simulink model "CD2_Library"  (Simulink 8.6)
settings: Solver=FixedStepDiscrete  StartTime=0  StopTime=7200  FixedStep=300  RelTol=1e-3
InitFcn:
  | CD2_init
undefined symbols (not defined in the file): CD2_get_substance_count, CD2_get_substances_count, Crain, get_blocks_id, input_c, subs_vect, table, tablestep
(part 1 of 2)
settings Model: Creator=garbanlo  LastModifiedBy=garbanlo
settings DataIOCC: LimitDataPoints=off  TimeSaveName=cd_time  SignalLoggingName=sigsOut
settings OptimizationCC: ExpressionDepthLimit=128  InitFltsAndDblsToZero=on
settings DebuggingCC: SaveWithParameterizedLinksMsg=none  SignalResolutionControl=TryResolveAllWithWarning  SolverPrmCheckMsg=none  MultiTaskDSMMsg=warning  MultiTaskCondExecSysMsg=none  FcnCallInpInsideContextMsg=UseLocalSettings  StateNameClashWarn=none  StrictBusMsg=None
settings HardwareCC: TargetUnknown=on
settings GRTTargetCC: TargetFcnLib=ansi_tfl_tmw.mat  GeneratePreprocessorConditionals=Use local settings

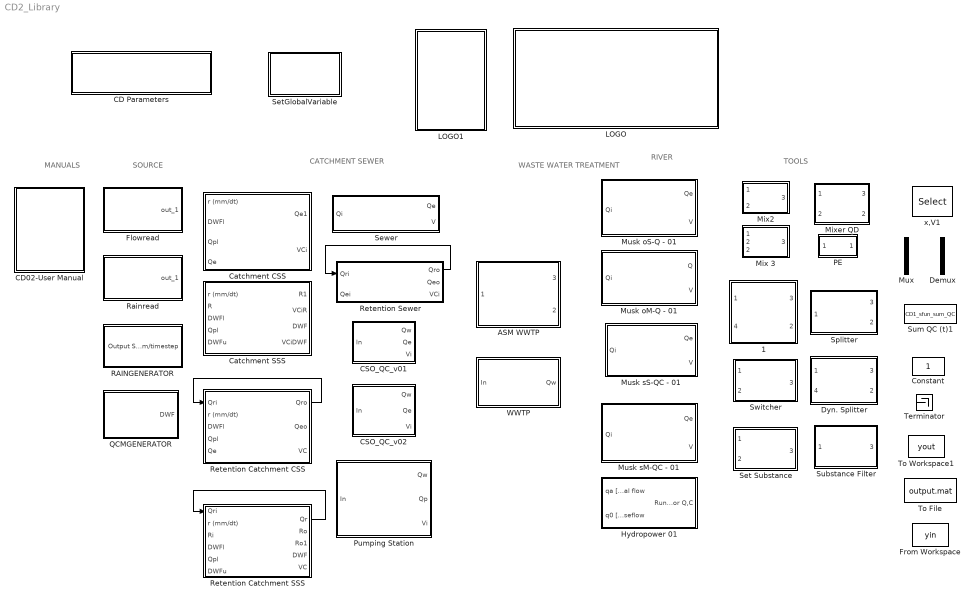
== system CD2_Library ==
  note: TOOLS
  note: SOURCE
  note: RIVER
  note: CATCHMENT
      | SEWER
  note: MANUALS
  note: WASTE WATER
      | TREATMENT
  " 1" : Subsystem  mask(Wrong Connect){n_comp=CD2_get_substances_count, values_rain=15, mode_rain=Percent [0-100], values_dwf=23, mode_dwf=Percent [0-100]}
      mask prompts: n_comp "Number of components"; values_rain "Fraction Qr --> Qdwf"; mode_rain "Splitting mode"; values_dwf "Fraction Qdwf --> Qr"; mode_dwf "Splitting mode"
      mask help: The block simulates wrong connections given in a seperate sewer system. MAgnitudes of wrong connections are described by fraction percentages (or quanities) diverted from or to the stormwater pipe.
      mask init:
      | % reading the toplevel systems' name 
      | % --> Plant file name;
      | tls=bdroot(gcb); 
      | % Obtaining the fixed sampling time
      | t_samp_char=get_param(tls, 'FixedStep');
      | % Convertion to numeric value
      | tstep = str2num(t_samp_char);
      mask TypeOptions mode_rain: Fraction [0-1] | Percent [0-100] | m³/s
      mask TypeOptions mode_dwf: Fraction [0-1] | Percent [0-100] | m³/s
      mask Display:
      | plot(0,0,100,100);
      | 
      | 
      | plot([30,70],[30,30]);
      | plot([30,70],[70,70]);
      | plot([40,60],[30,70]);
      | plot([40,60],[70,30]);
      | 
      | 
      | 
      | 
      | text(50,10,'WRONG Connect','HorizontalAlignment','center');
      | port_label('input',1,'Qr');
      | port_label('input',2,'Qdwf');
      | port_label('output',1,'Qr');
      | port_label('output',2,'Qdwf');
  " Dyn. Splitter" : Subsystem  mask(Splitter){n_comp=CD2_get_substances_count, mode=Percent [0-100]}
      mask prompts: n_comp "Number of components"; mode "Splitting mode"
      mask help: Splitter parameter.
      mask init: same as CD2_Library/ 1
      mask Help: Splits stream in 2 streams. Split by percent or by value.
      mask TypeOptions mode: Fraction [0-1] | Percent [0-100] | m³/s
      mask Display:
      | plot(0,0,100,100);
      | 
      | plot([30,50],[50,50]);
      | plot([50,70],[50,70]);
      | plot([50,70],[50,30]);
      | 
      | text(50,10,'Dyn. SPLITTER','HorizontalAlignment','center');
      | port_label('input',1,'Qi');
      | port_label('output',1,'Q1');
      | port_label('output',2,'Q2');
  " Hydropower 01" : Subsystem  mask(HYDROPOWER){n_comp=CD2_get_substances_count, C_Stream=[1 2 3]}
      mask prompts: n_comp "No of components"; C_Stream "Vector of Stream-Conc. g/m3"
      mask help:
      | Hydropower block for modelling downstream release of water. Upstream concnetration of baseflow ( qo ) and additional flow ( qa ) are considered constant.
      |
      | Used function:
      | CD1_sfun_hydropower
      mask init:
      | % reading the toplevel systems' name 
      | % --> Plant file name;
      | tls=bdroot(gcb); 
      | % Obtaining the fixed sampling time
      | t_samp_char=get_param(tls, 'FixedStep');
      | % Convertion to numeric value
      | tstep = str2num(t_samp_char);
      mask Display:
      | plot(0,0,100,100, [30 30 32 34 36 38 40 44 46 50], [28 60 62 65 67 70 70 67 65 25], [15 80],[30 20], [30 50],[34 30],[30 50],[38 34], [15 33],[65 65], [50 80],[45 40] );
      | text(50,90,'HYDROPOWER','HorizontalAlignment','center');
      | text(50,10,'baseflow','HorizontalAlignment','center');
      | port_label('input',1,'qa');
      | port_label('input',2,'qo');
      | port_label('output',1,'Qe');
  " Mixer QD" : Subsystem  mask(Mixer QD){n_comp=CD2_get_substances_count, Cmcl=[3 3 3]}
      mask prompts: n_comp "Number of pollutants [ - ]"; Cmcl "MCL - Vector of max. concentration limits [g/m3]"
      mask help:
      | Performes mixing of pollutant fluxes Qw  and Qo in accordance to their hydraulic load. Qo is considered to be the less pollluted flux. In addition the required increase of Qo is calculated for meeting required MCL (maximum concentration limits) defined by user input.
      |
      | Function used:
      | CD1_sfun_mixing_QC_QD.m
      mask init: same as CD2_Library/ 1
      mask Display:
      | plot(0,0,100,100);
      | 
      | text(50,60,'Mixing','HorizontalAlignment','center');
      | text(50,35,'QD','HorizontalAlignment','center');
      | 
      | 
      | port_label('input',1,'Qw');
      | port_label('input',2,'Qo');
      | port_label('output',1,'Qe');
      | port_label('output',2,'QD');
  ASM WWTP : Subsystem  mask(ASM WWTP){wwtpfile='wwtp_vils.txt', dtwwtp=30, frac=[1 1 1], n_comp=CD2_get_substances_count}
      mask prompts: wwtpfile "WWTP File"; dtwwtp "delta t WWTP"; frac "Fraction sol [0-1]"; n_comp "Number of pollutants [ - ]"
      mask help: WWTP unit that includes primray clarifier, biology and secondary clarifier. Biochemical modelling is based on a simplified ASM1 model.
      mask init: same as CD2_Library/ 1
      mask Display:
      | plot(0,0,100,100);
      | 
      | plot(0,0,100,100);
      | 
      | patch( [15,35,25,15],[55,55,30,55],[.6 0.6 .3]);
      | patch( [40,60,60,40,40],[30,30,55,55,30],[.8 0.6 .3]);
      | patch( [65,85,75,65],[55,55,30,55],[1 0.6 .3]);
      | 
      | plot( [15,35,25,15],[55,55,30,55], [30, 40],[40,40], [40,60,60,40,40],[30,30,55,55,30], [65,85,75,65],[55,55,30,55], [60, 70],[40,40] );
      | 
      | 
      | 
      | text(50,70,'ASM-WWTP','HorizontalAlignment','center');
      | 
      | 
      | port_label('input',1,'Qi');
      | port_label('output',1,'Qe');
      | port_label('output',2,'ASM1+P');
  CD Parameters : Subsystem  mask(City Drain 2.0 - Simulation parameters){subst='HCO3 NH4', t_step=300, t_start=0, t_stop=7200}
      mask prompts: subst "Modell Substances list (string)"; t_step "Sampling Time [s]"; t_start "Start Time [s]"; t_stop "Stop Time [s]"
      mask help:
      | Block that sets the global parameters required in City Drain 2.0. Following paramters are set without user's input:
      |
      | - 'Solver' --> 'FixedStepDiscrete'
      | - 'TimeSaveName' --> 'cd_time'
      | - 'Decimation' --> '1'
      | - 'LimitDataPoints' -->  'off'
      mask init:
      | % toplevel systems' name --> Plant file name;
      | tls=bdroot(gcb); 
      | set_param(tls, 'Solver', 'FixedStepDiscrete'); 
      | set_param(tls, 'TimeSaveName', 'cd_time');
      | set_param(tls, 'Decimation', '1');
      | set_param(tls, 'LimitDataPoints', 'off');
      | set_param(tls, 'ScreenColor', 'white');
      | 
      | tstep_char=num2str(t_step); % Setting the discrete time step
      | set_param(tls, 'FixedStep', tstep_char); 
      | 
      | tstart_char=num2str(t_start); % Setting the start time
      | set_param(tls, 'StartTime', tstart_char); 
      | 
      | tstop_char=num2str(t_stop); % Setting the stop time
      | set_param(tls, 'StopTime', tstop_char);
      | 
      | set_param(gcs,'InitFcn','CD2_init');
      mask Display:
      | plot(0,0,100,100);
      | 
      | text(50,65,'CITY DRAIN','HorizontalAlignment','center');
      | text(50,35,'PARAMETERS','HorizontalAlignment','center');
      | 
      | 
      | image(imread('CityDrain_SimParam.jpg'))
  CD02-User Manual : Subsystem  mask(Open Usermanual){}
      settings: OpenFcn=open('CD2_UserManual_2007.pdf');
      mask Display:
      | text(50,70,'CITY DRAIN 1.0','HorizontalAlignment','center');
      | text(50,40,'User Manual','HorizontalAlignment','center');
      | image(imread('CD1_start_user_manual.jpg'));
  CSO_QC_v01 : Subsystem  mask(CSO Typ A - Combined sewer overflow){Vmax=300, Qemax=0.1, n_comp=CD2_get_substances_count}
      mask prompts: Vmax "Basin Volume [m3]"; Qemax "Maximum Effluent flow [m3/s]"; n_comp "Number of Pollutants [-]"
      mask help:
      | Combined sewer overflow structure.
      | Diverts the inflow given into effluent and overflow. The model implemented consideres hydraulics and pollutant routing by full mixing in the structure.
      |
      | Function used:
      | CD1_sfun_cso_A.m
      mask init: same as CD2_Library/ 1
      mask Display:
      | plot(0,0,100,100);
      | 
      | text(50,60,'CSO','HorizontalAlignment','center');
      | text(50,30,'Typ A','HorizontalAlignment','center');
      | 
      | 
      | port_label('input',1,'Qi');
      | port_label('output',1,'Qw');
      | port_label('output',2,'Qe');
      | port_label('output',3,'Vi');
  CSO_QC_v02 : Subsystem  mask(CSO Typ B - Combined sewer overflow){Vmax=300, Qemax=0.1, n_comp=CD2_get_substances_count, n_sed=[0.2]}
      mask prompts: Vmax "Basin Volume (m3)"; Qemax "Maximum Effluent flow [m3/s]"; n_comp "Number of Pollutants [-]"; n_sed "n-sed (Vect. of Sed. Coefficients)"
      mask help:
      | Combined sewer overflow structure.
      | Diverts the inflow given into effluent and overflow. The model implemented consideres hydraulics and pollutant routing by full mixing in the structure.
      |
      | In addition to Type A a retenetion/sedimentation factor is introduced. The factor may be used for applying different ratios in pollutant concentration for effluent flow (QE) and overflow (QW).
      |
      | Function used:
      | CD1_sfun_cso_B.m
      mask init: same as CD2_Library/ 1
      mask Display:
      | plot(0,0,100,100);
      | 
      | 
      | text(50,60,'CSO','HorizontalAlignment','center');
      | text(50,30,'Typ B','HorizontalAlignment','center');
      | 
      | 
      | port_label('input',1,'Qi');
      | port_label('output',1,'Qw');
      | port_label('output',2,'Qe');
      | port_label('output',3,'Vi');
  Catchment CSS : Subsystem  mask(Catchment CSS){area=208, rfcoeff=0.20, initloss=1, permloss=1.25, N=3, n_comp=CD2_get_substances_count, Rain_C=1, K=300, X=0}
      mask prompts: area "Area in [ha]"; rfcoeff "Runoff coefficient (0 - 1)"; initloss "Initial Loss in [mm]"; permloss "Permanent loss in [mm/day]"; N "No of Timesteps (transport time) / No of subareas n [-]"; n_comp "No of pollutant components"; Rain_C "Vector of Rain-Conc. [g/m3]"
      mask help:
      | Hydrological model of an urban catchment with a combined sewer system.
      | --> see manual for more details
      mask init:
      | % location of catchment drawing
      | x=10;
      | y=-10;
      | % reading the toplevel systems' name 
      | % --> Plant file name;
      | tls=bdroot(gcb); 
      | % Obtaining the fixed sampling time
      | t_samp_char=get_param(tls, 'FixedStep');
      | % Convertion to numeric value
      | tstep = str2num(t_samp_char); 
      | 
      | %convertion form mm/day --> mm/DT
      | permloss=permloss/86400*tstep;
      | area=area*10000;
      | 
      | %parameter for muskingum
      | CX=(tstep/2-K*X)/(tstep/2+K*(1-X));
      | CY=1/(tstep/2+K*(1-X));
      mask Display:
      | plot(0,0,100,100, [17 20 25 30 40 45 50 55 60 65]+x, [60 80 82 85 88 88 88 85 75 60]+y);
      | plot(0,0,100,100, [17 20 25 30 40 45 50 55 60 65]+x, [55 40 35 30 30 30 30 35 40 55]+y);
      | 
      | plot([20 65]+x,[60 60]+y);
      | plot([20 30]+x,[80 60]+y);
      | plot([30 40]+x,[75 60]+y);
      | plot([45 60]+x,[75 60]+y);
      | plot([20 65]+x,[55 55]+y);
      | plot([20 30]+x,[40 55]+y);
      | plot([30 40]+x,[45 55]+y);
      | plot([45 60]+x,[30 55]+y);
      | 
      | color('black');
      | 
      | port_label('input',1,'rl');
      | port_label('input',2,'DWFl');
      | port_label('input',3,'Qpl');
      | port_label('input',4,'Qe');
      | port_label('output',1,'Qe');
      | port_label('output',2,'VCi');
      | 
      | text(50,90,'CATCHMENT CSS','HorizontalAlignment','center');
  Catchment SSS : Subsystem  mask(Catchment SSS){area=27, rfcoeff=0.16, initloss=1, permloss=1.25, N=6, n_comp=CD2_get_substances_count, Rain_C=1, K=300, X=0}
      mask prompts: area "Area in [ha]"; rfcoeff "Runoff coefficient (0 - 1)"; initloss "Initial Loss in [mm]"; permloss "Permanent loss in [mm/day]"; N "No of Timesteps (transport time) / No of subareas n [-]"; n_comp "No of pollutant components"; Rain_C "Vector of Rain-Conc. [g/m3]"
      mask help:
      | Hydrological model of an urban catchment with a separate sewer system.
      | --> see manual for more details
      mask init: same as CD2_Library/Catchment CSS
      mask Display:
      | plot(0,0,100,100, [17 20 25 30 40 50 55 60 70 75 80]+x, [60 80 82 85 88 88 88 85 82 75 60]+y);
      | 
      | plot([20 80]+x,[60 60]+y);
      | plot([20 30]+x,[80 60]+y);
      | plot([30 40]+x,[75 60]+y);
      | plot([45 60]+x,[75 60]+y);
      | 
      | color('white');
      | plot([20 80]+x,[55 55]+y);
      | plot([20 30]+x,[40 55]+y);
      | plot([30 40]+x,[45 55]+y);
      | plot([45 60]+x,[30 55]+y);
      | 
      | color('black');
      | 
      | port_label('input',1,'rl');
      | port_label('input',2,'R');
      | port_label('input',3,'DWFl');
      | port_label('input',4,'Qpl');
      | port_label('input',5,'DWFu');
      | port_label('output',1,'R');
      | port_label('output',2,'VCi(R)');
      | port_label('output',3,'DWF');
      | port_label('output',4,'VCi(DWF)');
      | 
      | 
      | text(50,90,'CATCHMENT SSS','HorizontalAlignment','center');
  Constant : Constant
  Demux : Demux  Outputs=[13,1]
  Flowread : Subsystem  mask(CD1_Flowread){table0='Input_CSO_QC_Test_01.txt', dtype=Composite sample, crep=off}
      mask prompts: table0 "Filename"; dtype "Data type"; crep "Cylic repitition"
      mask help:
      | Reads flowdata (Q) and substance concentration (Ci) associated from ascii file.
      |
      | Used function:
      | CD1_sfun_flowread.m
      | CD1_mfun_flowread.m
      mask init:
      | table=CD1_mfun_flowread(table0);
      | 
      | 
      | % reading the toplevel systems' name 
      | % --> Plant file name;
      | tls=bdroot(gcb); 
      | % Obtaining the fixed sampling time
      | t_samp_char=get_param(tls, 'FixedStep');
      | % Convertion to numeric value
      | tstep = str2num(t_samp_char);
      mask TypeOptions dtype: Composite sample | Grab sample
      mask Display:
      | plot(0,0,100,100);
      | 
      | text(50,20,'FLOWREAD','HorizontalAlignment','center');
      | 
      | plot( [5 10 10 15 15 20 20 25 25 30 30 35 35 40], [0 0 10 10 20 20 40 40 20 20 0 0 0 0]+50);
      | plot( [5 10 15 20 25 30 35 ]+50, [0 5 10 15 30 20 0]+50);
  From Workspace : FromWorkspace  VariableName=yin  OutputAfterFinalValue=Setting to zero
  LOGO : Subsystem  mask(LOGO CITY DRAIN){}
      mask help:
      | Displays the City Drain Logo in Color
      |
      | Source file:
      | CityDrainLogo_C1.jpg
      mask Display: image(imread('CityDrain 2Logo_C1.jpg'));
  LOGO1 : Subsystem  mask(LOGO CITY DRAIN){}
      mask help:
      | Displays the City Drain Logo in Color
      |
      | Source file:
      | CityDrainLogo_C1.jpg
      mask Display: image(imread('LOGO_IUT4C.jpg'));
  Mix 3 : Subsystem  mask(Mixer){n_comp=CD2_get_substances_count}
      mask prompts: n_comp "Number of pollutants [ - ]"
      mask help:
      | Performes mixing of pollutant fluxes Q1 and Q2 in accordance to their hydraulic load.
      |
      | Function used:
      | CD1_sfun_mixing_QC.m
      mask init: same as CD2_Library/ 1
      mask Display:
      | plot(0,0,100,100);
      | 
      | text(50,50,'Mix3','HorizontalAlignment','center');
      | 
      | 
      | port_label('input',1,'Q1');
      | port_label('input',2,'Q2');
      | port_label('input',3,'Q3');
      | port_label('output',1,'Qe');
  Mix2 : Subsystem  mask(Mixer){n_comp=CD2_get_substances_count}
      mask prompts: n_comp "Number of pollutants [ - ]"
      mask help:
      | Performes mixing of pollutant fluxes Q1 and Q2 in accordance to their hydraulic load.
      |
      | Function used:
      | CD1_sfun_mixing_QC.m
      mask init: same as CD2_Library/ 1
      mask Display:
      | plot(0,0,100,100);
      | 
      | text(50,50,'Mix2','HorizontalAlignment','center');
      | 
      | 
      | port_label('input',1,'Q1');
      | port_label('input',2,'Q2');
      | port_label('output',1,'Qe');
  Musk oM-Q - 01 : Subsystem  mask(Muskingum - Cunge flood rooting (original scheme)){K=900, X=0.2, N=2}
      mask prompts: K "K (travel time of one subreach) [ s ]"; X "X (weighing factor) [ - ]"; N "N (Number of sub-reaches) [ - ]"
      mask help:
      | Flood routing using the original scheme by Muskingum-Cunge for multiple river stretches for hydraulic routing only.
      | The block accepts flow inputs and returns effluent fluxes and current stated of retained volume.
      | Intial Conditions: V=0; and Qe=0;
      |
      | Function used:
      | CD1_sfun_Muskingum_oM_Q.m
      mask init:
      | m=[5,5];%Offset for arrow 
      | l=[65,15];%Offset for arrow 
      | x=0; 
      | y=-15; %Offset for river
      | 
      | % reading the toplevel systems' name-> Plant file name;
      | tls=bdroot(gcb); 
      | % Obtaining the fixed sampling time
      | tstep_char=get_param(tls, 'FixedStep');
      | % Convertion to numeric value
      | dt = str2num(tstep_char); 
      | 
      | 
      | 
      | %Muskingum parameters
      | D=K.*(1-X)+0.5.*dt;
      | C0=(0.5.*dt-K.*X)./D;
      | C1=(0.5.*dt+K.*X)./D;
      | C2=(K.*(1-X)-0.5.*dt)./D;
      mask Display:
      | plot(0,0,100,100, [20,30,40,50,60,70,80]+x, [35,40,45,50,45,40,45]+y, [20,30,40,50,60,70,80]+x, [75,85,90,95,90,85,90]+y, [30,30]+x,[40,85]+y, [50,50]+x,[50,95]+y, [70,70]+x,[40,85]+y );
      | 
      | plot( [10,10,15,15,20,15,15,10]+m(1), [40,30,30,22,35,48,40,40]+m(2), [10,10,15,15,20,15,15,10]+l(1), [40,30,30,22,35,48,40,40]+l(2) );
      | 
      | text(40+x,65+y,'j');
      | text(55+x,65+y,'j+1');
      | 
      | text(50,90,'river q','HorizontalAlignment','center');
      | text(50,10,'muskingum-oM-Q','HorizontalAlignment','center');
      | 
      | port_label('input',1,'qi');
      | port_label('output',1,'qe');
      | port_label('output',2,'v');
  Musk oS-Q - 01 : Subsystem  mask(Muskingum - Cunge flood rooting (original scheme)){K=300, X=0.2}
      mask prompts: K "K (travel time of the reach) [s]"; X "X (weighing factor)  [ - ]"
      mask help:
      | Flood routing unsing the original scheme by Muskingum-Cunge for a single river stretch for hydraulic routing only.
      | The block accepts flow inputs and returns effluent fluxes and current stated of retained volume.
      | Intial Conditions: V=0; and Qe=0;
      |
      | Function used:
      | CD1_sfun_Muskingum_oS_Q.m
      mask init:
      | % reading the toplevel systems' name 
      | % --> Plant file name;
      | tls=bdroot(gcb); 
      | % Obtaining the fixed sampling time
      | t_samp_char=get_param(tls, 'FixedStep');
      | % Convertion to numeric value
      | dt = str2num(t_samp_char); 
      | 
      | %Muskingum parameters
      | D=K.*(1-X)+0.5.*dt;
      | C0=(0.5.*dt-K.*X)./D;
      | C1=(0.5.*dt+K.*X)./D;
      | C2=(K.*(1-X)-0.5.*dt)./D;
      mask Display:
      | plot(0,0,100,100, [20,80],[30,20],[20,80],[80,50], [20,20],[30,80],[80,80],[20,50], [15,27],[55,50],[24,27,24,24],[53,50,48,53], [75,87],[35,30],[84,87,84,84],[33,30,28,33])
      | plot([20,80],[60,50])
      | 
      | text(50,40,'V');
      | text(50,90,'river q','HorizontalAlignment','center');
      | text(50,10,'muskingum-oS-Q','HorizontalAlignment','center');
      | 
      | port_label('input',1,'qi');
      | port_label('output',1,'qe');
      | port_label('output',2,'v');
  Musk sM-QC - 01 : Subsystem  mask(Muskingum - Cunge flood rooting - simplified scheme){K=300, X=0.3, n_comp=CD2_get_substances_count, N=1}
      mask prompts: K "K (travel time of a subreach) [s]"; X "X (weighing factor)  [ - ]"; n_comp "Number of pollutants [ - ]"; N "N (Number of sub-reaches) [ - ]"
      mask help:
      | Flood routing using the Muskingum-Cunge scheme for multiple river stretches for hydraulic and pollutant routing.
      | The block accepts flow inputs and returns effluent fluxes and current stated of retained volume.
      | Intial Conditions: V=0; and Qe=0;
      |
      | Function used:
      | CD1_sfun_Muskingum_sM_QC.m
      mask init:
      | m=[5,5];%Offset for arrow 
      | l=[65,15];%Offset for arrow 
      | x=0; 
      | y=-15; %Offset for river
      | 
      | % reading the toplevel systems' name 
      | % --> Plant file name;
      | tls=bdroot(gcb); 
      | % Obtaining the fixed sampling time
      | t_samp_char=get_param(tls, 'FixedStep');
      | % Convertion to numeric value
      | dt = str2num(t_samp_char); 
      | 
      | %Muskingum parameters
      | CA=0.5.*dt-K.*X;
      | CB=0.5.*dt+K.*(1-X);
      mask Display:
      | plot(0,0,100,100, [20,30,40,50,60,70,80]+x, [35,40,45,50,45,40,45]+y, [20,30,40,50,60,70,80]+x, [75,85,90,95,90,85,90]+y, [30,30]+x,[40,85]+y, [50,50]+x,[50,95]+y, [70,70]+x,[40,85]+y );
      | 
      | plot( [10,10,15,15,20,15,15,10]+m(1), [40,30,30,22,35,48,40,40]+m(2), [10,10,15,15,20,15,15,10]+l(1), [40,30,30,22,35,48,40,40]+l(2) );
      | 
      | text(40+x,65+y,'j');
      | text(55+x,65+y,'j+1');
      | 
      | text(50,90,'RIVER QC','HorizontalAlignment','center');
      | text(50,10,'MUSKINGUM-sM-QC','HorizontalAlignment','center');
      | 
      | port_label('input',1,'Qi');
      | port_label('output',1,'Qe');
      | port_label('output',2,'V');
  Musk sS-QC - 01 : Subsystem  mask(Muskingum - Cunge flood rooting){K=300, X=0.2, n_comp=CD2_get_substances_count}
      mask prompts: K "K (travel time of the reach) [s]"; X "X (weighing factor)  [ - ]"; n_comp "Number of pollutants n [ - ]"
      mask help:
      | Flood routing using the Muskingum-Cunge scheme for a single river stretch. Routing is provide for hydraulics and pollutants using a simplified discrete scheme.
      | The block accepts flow inputs and returns effluent fluxes and current states of retained volume.
      | Intial Conditions: V=0; and Qe=0;
      |
      | Function used:
      | CD1_sfun_Muskingum_sS_QC.m
      mask init:
      | % reading the toplevel systems' name 
      | % --> Plant file name;
      | tls=bdroot(gcb); 
      | % Obtaining the fixed sampling time
      | t_samp_char=get_param(tls, 'FixedStep');
      | % Convertion to numeric value
      | dt = str2num(t_samp_char); 
      | 
      | %Muskingum parameters
      | CA=0.5.*dt-K.*X;
      | CB=0.5.*dt+K.*(1-X);
      mask Display:
      | plot(0,0,100,100, [20,80],[30,20],[20,80],[80,50], [20,20],[30,80],[80,80],[20,50], [15,27],[55,50],[24,27,24,24],[53,50,48,53], [75,87],[35,30],[84,87,84,84],[33,30,28,33]);
      | plot([20,80],[60,50])
      | 
      | 
      | text(50,40,'V');
      | 
      | text(50,90,'RIVER QC','HorizontalAlignment','center');
      | text(50,10,'MUSKINGUM sS-QC','HorizontalAlignment','center');
      | 
      | port_label('input',1,'Qi');
      | port_label('output',1,'Qe');
      | port_label('output',2,'V');
  Mux : Mux  Inputs=[13,1]
  PE : Subsystem  mask(Inhabitants){EG=1000}
      mask help: Multiply source with inhabitants.
      mask init:
      | % reading the toplevel systems' name 
      | % --> Plant file name;
      | tls=bdroot(gcb); 
      | % Obtaining the fixed sampling time
      | t_samp_char=get_param(tls, 'FixedStep');
      | % Convertion to numeric value
      | t_step = str2num(t_samp_char);
      mask Display:
      | plot(0,0,100,100);
      | 
      | text(30,45,'PE');
  Pumping Station : Subsystem  mask(Pumping Station){Vmax=100, NP=1, Qp=[0.031], Von=[18.5], Voff=[0], n_comp=CD2_get_substances_count}
      mask prompts: Vmax "Basin Volume [m3]"; NP "NP - Number of pumps"; Qp "Qp - Pumping rates [m3/s]"; Von "Von  - ON - set points for pumps"; Voff "Voff - OFF - set points for pumps"; n_comp "Number of Pollutants [-]"
      mask help:
      | A pumping station base on a discrete numerical scheme
      |
      | Function used:
      | CD1_sfun_pump_A.m
      mask init:
      | % reading the toplevel systems' name 
      | % --> Plant file name;
      | tls=bdroot(gcb); 
      | % Obtaining the fixed sampling time
      | t_samp_char=get_param(tls, 'FixedStep');
      | % Convertion to numeric value
      | tstep = str2num(t_samp_char); 
      | 
      | %PLOTTING
      | mx=60;
      | my=40;
      | spump=5;
      | sarrow=2;
      | 
      | 
      | p=0:pi/2/2:2*pi; 
      | x=cos(p).*spump+mx; 
      | y=sin(p).*spump+my;
      | 
      | p2=0:pi.*2/3:2*pi; p2=p2+pi/2; 
      | a=cos(p2).*spump+mx; 
      | b=sin(p2).*spump+my; 
      | 
      | p3=0:pi.*2/3:2*pi;  
      | c=cos(p3).*sarrow; 
      | d=sin(p3).*sarrow;
      mask Display:
      | plot(0,0,100,100);
      | 
      | text(50,20,'Pumping Station','HorizontalAlignment','center');
      | 
      | 
      | patch([30 30 70 70], [60 30 30 60],[1 0.7 0]);
      | 
      | plot([29 29 71 71], [80 29 29 80]);
      | plot([28 28 72 72], [80 28 28 80]);
      | 
      | plot(x,y); patch(x,y,[1 1 1]); patch(a,b,[0 0 0]);
      | plot([0 0 20]+mx, [0 10 10]+my);
      | patch(c+mx+20,d+my+10,[0 0 0]);
      | 
      | port_label('input',1,'Qi');
      | port_label('output',1,'Qw');
      | port_label('output',2,'Qp');
      | port_label('output',3,'Vi');
  QCMGENERATOR : Subsystem  mask(QCM Generator){yi1=[1 0.32 0.32 0.32 0.32 0.32 0.32 1 1 1 1.7 1.7 1.4 0.9 1 1 1.7 1.7 1 1 1 1 1 1 1], xi1=[0 1 2 3 4 5 6 7 8 9 10 11 12 13 14 15 16 17 18 19 20 21 22 23 24], ewg1=488, yi2=[1 0.32 0.32 0.32 0.32 0.32 0.32 1 1 1 1.7 1.7 1.4 0.9 1 1 1.7 1.7 1 1 1 1 1 1 1], xi2=[0 1 2 3 4 5 6 7 8 9 10 11 12 13 14 15 16 17 18 19 20 21 22 23 24], ewg2=488, itype='linear'}
      mask prompts: yi1 "Workdays Q/m/c [m3/s;m3;g/m3]"; xi1 "Workdays time [s]"; ewg1 "Workdays daily mean [m3/s;m3;g/m3]"; yi2 "Weekends Q/m/c [m3/s;m3;g/m3]"; xi2 "Weekends time [s]"; ewg2 "Weekends daily mean [m3/s;m3;g/m3]"; itype "Interpolations type"
      mask help:
      | Generates either one of
      | - Q ...flows [m3/s]
      | - C ...Concentration [g/m3]
      | - M ...Massflux [g/s]
      mask init:
      | tls=bdroot(gcb); 
      | t_samp_char=get_param(tls, 'FixedStep');
      | tstep = str2num(t_samp_char);
      | % Create Spline for Mo-Fr
      | 
      | 
      | [y,ye] = CD1_mfun_graph_generator(xi1,yi1,xi2,yi2,itype,ewg1,ewg2,tstep);
      | yy=y.*tstep.*86400./tstep;
      | yye=ye.*tstep.*86400./tstep;
      mask Display:
      | plot(0,0,100,100);
      | 
      | text(60,40,'QCM');
      | text(20,10,'GENERATOR');
      | 
      | plot([4 4],[20 40]);
      | plot([6 6],[20 30]);
      | plot([8 8],[20 35]);
      | plot([10 10],[20 50]);
      | plot([12 12],[20 55]);
      | plot([14 14],[20 20]);
      | plot([16 16],[20 22]);
      | plot([18 18],[20 22]);
      | plot([20 20],[20 45]);
      | plot([22 22],[20 50]);
      | plot([24 24],[20 20]);
      | plot([26 26],[20 20]);
      | plot([28 28],[20 20]);
      | plot([30 30],[20 60]);
  RAINGENERATOR : Subsystem  mask(Rain Generator){param=[1,3,0.2,0.3]}
      mask prompts: param "Parameters [a,b,c,d]"
      mask help: Generates rain pattern by means of stochstics.
      mask init:
      | a=param(1);
      | b=param(2);
      | c=param(3);
      | d=param(4);
      | 
      | % reading the toplevel systems' name 
      | % --> Plant file name;
      | tls=bdroot(gcb); 
      | % Obtaining the fixed sampling time
      | t_samp_char=get_param(tls, 'FixedStep');
      | % Convertion to numeric value
      | t_step = str2num(t_samp_char);
      mask Display:
      | plot(0,0,100,100);
      | 
      | text(60,40,'RAIN');
      | text(20,10,'GENERATOR');
      | 
      | plot([4 4],[20 40]);
      | plot([6 6],[20 30]);
      | plot([8 8],[20 35]);
      | plot([10 10],[20 50]);
      | plot([12 12],[20 55]);
      | plot([14 14],[20 20]);
      | plot([16 16],[20 22]);
      | plot([18 18],[20 22]);
      | plot([20 20],[20 45]);
      | plot([22 22],[20 50]);
      | plot([24 24],[20 20]);
      | plot([26 26],[20 20]);
      | plot([28 28],[20 20]);
      | plot([30 30],[20 60]);
  Rainread : Subsystem  mask(Rain Read){table0='test2.km2', crep=off}
      mask prompts: table0 "Filename"; crep "Cylic repitition"
      mask help:
      | Read raindata from ASCII File in following formats:
      |
      | *.ixx ... Format used by the Austrian Hydrographic Service.
      | *.km2 ... Format used in the Mouse Software from DHI (Danish Hydraulic Institute)
      | *.mse ... modified mse format used in  Mouse Software from DHI (Danish Hydraulic Institute)
      |
      | Used function: CD1_mfun_rainread.m
      mask init:
      | % cache table size set to 1000
      | %table=zeros(1000,2)
      | [table,tablestep]=CD1_mfun_rainread(table0);
      | 
      | % reading the toplevel systems' name 
      | % --> Plant file name;
      | tls=bdroot(gcb); 
      | % Obtaining the fixed sampling time
      | t_samp_char=get_param(tls, 'FixedStep');
      | % Convertion to numeric value
      | tstep = str2num(t_samp_char);
      mask Display:
      | plot(0,0,100,100);
      | 
      | text(40,40,'RAIN READ');
      | plot( [5 10 10 15 15 20 20 25 25 30 30 40 40 45], [0 0 20 20 40 40 60 60 30 30 0 0 0 0]+20);
  Retention Catchment CSS : Subsystem  mask(Retention Catchment CSS){area=208, rfcoeff=0.20, initloss=1, permloss=1.25, N=3, n_comp=CD2_get_substances_count, Rain_C=1, K=300, X=0, Vsmax=100, Qemax=0.4, n_sed=0}
      mask prompts: area "Area in [ha]"; rfcoeff "Runoff coefficient (0 - 1)"; initloss "Initial Loss in [mm]"; permloss "Permanent loss in [mm/day]"; N "No of Timesteps (transport time) / No of subareas n [-]"; n_comp "No of pollutant components"; Rain_C "Vector of Rain-Conc. [g/m3]"; Vsmax "Storage volume [m3]"; Qemax "Maxiumum effluent flow [m3/s]"; n_sed "n-sed (Vect. of Sed. Coefficients)"
      mask help:
      | Hydrological model of an urban catchment with a combined sewer system.
      | Including additional retention of fluxes to mimic storage.
      | --> see manual for more details
      mask init:
      | % location of catchment drawing
      | x=10;
      | y=-10;
      | % reading the toplevel systems' name 
      | % --> Plant file name;
      | tls=bdroot(gcb); 
      | % Obtaining the fixed sampling time
      | t_samp_char=get_param(tls, 'FixedStep');
      | % Convertion to numeric value
      | tstep = str2num(t_samp_char);
      mask Display:
      | plot(0,0,100,100, [17 20 25 30 40 45 50 55 60 65]+x, [60 80 82 85 88 88 88 85 75 60]+y);
      | plot(0,0,100,100, [17 20 25 30 40 45 50 55 60 65]+x, [55 40 35 30 30 30 30 35 40 55]+y);
      | 
      | plot([20 65]+x,[60 60]+y);
      | plot([20 30]+x,[80 60]+y);
      | plot([30 40]+x,[75 60]+y);
      | plot([45 60]+x,[75 60]+y);
      | plot([20 65]+x,[55 55]+y);
      | plot([20 30]+x,[40 55]+y);
      | plot([30 40]+x,[45 55]+y);
      | plot([45 60]+x,[30 55]+y);
      | 
      | color('black');
      | 
      | port_label('input',1,'Qr');
      | port_label('input',2,'rl');
      | port_label('input',3,'DWFl');
      | port_label('input',4,'Qpl');
      | port_label('input',5,'Qe');
      | port_label('output',1,'Qr');
      | port_label('output',2,'Qe');
      | port_label('output',3,'Vi');
      | 
      | text(50,90,'CATCHMENT CSS s','HorizontalAlignment','center');
  Retention Catchment SSS : Subsystem  mask(Retention Catchment SSS){area=input_c(1,get_blocks_id), rfcoeff=input_c(2,get_blocks_id), initloss=input_c(3,get_blocks_id), permloss=input_c(4,get_blocks_id), N=input_c(5,get_blocks_id), n_comp=CD2_get_substances_count, Rain_C=input_c(6,get_blocks_id), K=300, X=input_c(7,get_blocks_id), Vsmax=input_c(8,get_blocks_id), Qemax=input_c(9,get_blocks_id), n_sed=0}
      mask prompts: area "Area in [ha]"; rfcoeff "Runoff coefficient (0 - 1)"; initloss "Initial Loss in [mm]"; permloss "Permanent loss in [mm/day]"; N "No of Timesteps (transport time) / No of subareas n [-]"; n_comp "No of pollutant components"; Rain_C "Vector of Rain-Conc. [g/m3]"; Vsmax "Storage volume [m3]"; Qemax "Maxiumum effluent flow [m3/s]"; n_sed "n-sed (Vect. of Sed. Coefficients)"
      mask help:
      | Hydrological model of an urban catchment with a separate sewer system.
      | Including additional retention of fluxes to mimic storage.
      | --> see manual for more details
      mask init:
      | % location of catchment drawing
      | x=10;
      | y=-10;
      | % reading the toplevel systems' name 
      | % --> Plant file name;
      | tls=bdroot(gcb); 
      | % Obtaining the fixed sampling time
      | t_samp_char=get_param(tls, 'FixedStep');
      | % Convertion to numeric value
      | tstep = str2num(t_samp_char);
      mask Display:
      | plot(0,0,100,100, [17 20 25 30 40 50 55 60 70 75 80]+x, [60 80 82 85 88 88 88 85 82 75 60]+y);
      | 
      | plot([20 80]+x,[60 60]+y);
      | plot([20 30]+x,[80 60]+y);
      | plot([30 40]+x,[75 60]+y);
      | plot([45 60]+x,[75 60]+y);
      | 
      | color('white');
      | plot([20 80]+x,[55 55]+y);
      | plot([20 30]+x,[40 55]+y);
      | plot([30 40]+x,[45 55]+y);
      | plot([45 60]+x,[30 55]+y);
      | 
      | color('black');
      | 
      | port_label('input',1,'Qr');
      | port_label('input',2,'rl');
      | port_label('input',3,'R');
      | port_label('input',4,'DWFl');
      | port_label('input',5,'Qpl');
      | port_label('input',6,'DWFu');
      | port_label('output',1,'Qr');
      | port_label('output',2,'R');
      | port_label('output',3,'VCi(R)');
      | port_label('output',4,'DWF');
      | port_label('output',5,'VCi(DWF)');
      | 
      | 
      | 
      | text(50,90,'CATCHMENT SSS s','HorizontalAlignment','center');
  Retention Sewer : Subsystem  mask(Retention Sewer){K=300, X=0.1, n_comp=CD2_get_substances_count, N=11, Vsmax=100, Qemax=0.18, n_sed=0}
      mask prompts: K "K (travel time of a subreach) [s]"; X "X (weighing factor)  [ - ]"; n_comp "Number of pollutants [ - ]"; N "Number of sub-reaches [ - ]"; Vsmax "Storage volume [m3]"; Qemax "Maximum effluent flow [m3/s]"; n_sed "n-sed (Vect. of Sed. Coefficients)"
      mask help:
      | Function used:
      | CD1_sfun_Muskingum_Sewer.m
      mask init:
      | %arrow location in icon
      | kx=70;
      | ky=25;
      | % picture location
      | x=20;y=25;
      | 
      | 
      | % reading the toplevel systems' name 
      | % --> Plant file name;
      | tls=bdroot(gcb); 
      | % Obtaining the fixed sampling time
      | t_samp_char=get_param(tls, 'FixedStep');
      | % Convertion to numeric value
      | dt = str2num(t_samp_char);
      mask Display:
      | plot(0,0,100,50, [0,50,50,0,0]+x,[-10,-10,10,10,-10]+y, [10,10]+x,[-10,10]+y, [20,20]+x,[-10,10]+y, [30,30]+x,[-10,10]+y, [40,40]+x,[-10,10]+y, [0,0,5,5,10,5,5,0]+kx, [5,-5,-5,-13,0,13,5,5]+ky );
      | 
      | 
      | text(50,7,'SEWER sMS','HorizontalAlignment','center');
      | 
      | port_label('input',1,'Qr');
      | port_label('input',2,'Qe');
      | port_label('output',1,'Qr');
      | port_label('output',2,'Qe');
      | port_label('output',3,'VCi');
  Set Substance : Subsystem  mask(Set Q/C){subs_vect='Temp', n_comp=CD2_get_substances_count}
      mask prompts: subs_vect "Added substances vector"; n_comp "Number of pollutants [ - ]"
      mask help:
      | Set concentrations of pollutants and/or Q in flow.
      |
      | Function used:
      | CD2_sfun_mixing_QC_subs.m
      mask init: same as CD2_Library/ 1
      mask Display:
      | plot(0,0,100,100);
      | 
      | text(50,50,'Set Q/C','HorizontalAlignment','center');
      | 
      | 
      | port_label('input',1,'Q/C');
      | port_label('input',2,'Qi');
      | port_label('output',1,'Qe');
  SetGlobalVariable : Subsystem  mask(Set-Global-Param){Vname=Crain, Vvalue=[0 0 0 0 0.418 48/1000 81 1]}
      mask prompts: Vname "Variables names"; Vvalue "Variables values"
      mask help:
      | This block is designed to set a global parameter(variable) at the workspace, prior the simulation start.
      |
      | Setting is done after saving the current mdl-file.
      | BlockProperties -> Callbacks -> PostSaveFcn
      settings: AttributesFormatString="\"%<Vname>\""
      settings: PostSaveFcn=|
      | cb_name=get_param(gcb,'Vname');
      | cb_value=get_param(gcb,'Vvalue');
      | assignin('base',cb_name,str2num(cb_value));
      | clear('cb_value');
      | clear('cb_name');
      mask Display:
      | plot(0,0,100,100);
      | 
      | patch( [0,100,100,0,0],[50,50,100,100,50],[0 0.4 0.6]);
      | patch( [0,100,100,0,0],[0,0,50,50,0],[0 0.6 0.4]);
      | 
      | text(50,60,'Set','HorizontalAlignment','center');
      | text(50,30,'GlobalVar','HorizontalAlignment','center');
  Sewer : Subsystem  mask(Sewer){K=300, X=0.1, n_comp=CD2_get_substances_count, N=11}
      mask prompts: K "K (travel time of a subreach) [s]"; X "X (weighing factor)  [ - ]"; n_comp "Number of pollutants [ - ]"; N "N (Number of sub-reaches) [ - ]"
      mask help:
      | Function used:
      | CD1_sfun_Muskingum_Sewer.m
      mask init:
      | %arrow location in icon
      | kx=70;
      | ky=25;
      | % picture location
      | x=20;y=25;
      | 
      | 
      | % reading the toplevel systems' name 
      | % --> Plant file name;
      | tls=bdroot(gcb); 
      | % Obtaining the fixed sampling time
      | t_samp_char=get_param(tls, 'FixedStep');
      | % Convertion to numeric value
      | dt = str2num(t_samp_char); 
      | 
      | %Muskingum parameters
      | CA=0.5.*dt-K.*X;
      | CB=0.5.*dt+K.*(1-X);
      mask Display:
      | plot(0,0,100,50, [0,50,50,0,0]+x,[-10,-10,10,10,-10]+y, [10,10]+x,[-10,10]+y, [20,20]+x,[-10,10]+y, [30,30]+x,[-10,10]+y, [40,40]+x,[-10,10]+y, [0,0,5,5,10,5,5,0]+kx, [5,-5,-5,-13,0,13,5,5]+ky );
      | 
      | 
      | text(50,7,'SEWER sM','HorizontalAlignment','center');
      | 
      | port_label('input',1,'Qi');
      | port_label('output',1,'Qe');
      | port_label('output',2,'VCi');
  "Splitter " : Subsystem  mask(Splitter){n_comp=CD2_get_substances_count, values=40, mode=Percent [0-100]}
      mask prompts: n_comp "Number of components"; values "Fraction / Amount directed to Q1"; mode "Splitting mode"
      mask help: Splitter parameter.
      mask init: same as CD2_Library/ 1
      mask Help: Splits stream in 2 streams. Split by percent or by value.
      mask TypeOptions mode: Fraction [0-1] | Percent [0-100] | m³/s
      mask Display:
      | plot(0,0,100,100);
      | 
      | plot([30,50],[50,50]);
      | plot([50,70],[50,70]);
      | plot([50,70],[50,30]);
      | 
      | text(50,10,'SPLITTER','HorizontalAlignment','center');
      | port_label('input',1,'Qi');
      | port_label('output',1,'Q1');
      | port_label('output',2,'Q2');
  Substance Filter : Subsystem  mask(Filter){subs_vect='CO2 CO2', n_comp=CD2_get_substances_count}
      mask prompts: subs_vect "Added substances vector"; n_comp "Number of pollutants [ - ]"
      mask help:
      | Filters input for a set of element(Flow and concnetrations).
      |
      | Function used:
      | CD2_sfun_out_subs.m
      mask init: same as CD2_Library/ 1
      mask Display:
      | plot(0,0,100,100);
      | 
      | text(50,50,'Filter','HorizontalAlignment','center');
      | 
      | 
      | port_label('input',1,'Qi');
      | port_label('output',1,'S');
  Sum QC (t)1 : S-Function  FunctionName=CD1_sfun_sum_QC  Parameters=n_p, tstep  SFunctionDeploymentMode=off  EnableBusSupport=off  mask(Cumulation of Masses){n_p=1}
      mask prompts: n_p "Number of pollutants [ - ]"
      mask help:
      | This block returns the total hydraulic load V [m3] and the pollutant load M [g] during the simulation run.
      |
      | Function used:
      | CD1_sfun_sum_QC_t.m
      mask init: same as CD2_Library/ Hydropower 01
      mask Display:
      | plot(0,0,100,100);
      | text(50,50,'Sum QC(t)','HorizontalAlignment','center');
  Switcher : Subsystem  mask(Switcher){n_comp=CD2_get_substances_count, wechsler=0}
      mask prompts: n_comp "Number of pollutants [ - ]"; wechsler "Switch"
      mask help:
      | Switching of flows Q1 and Q2 in accordance the mask parameter switch.
      | Switch=1 => Q1
      | Switch=0 => Q2
      |
      | Function used:
      | CD1_sfun_switcher.m
      mask init: same as CD2_Library/ 1
      mask Display:
      | plot(0,0,100,100);
      | 
      | text(50,50,'SWITCH','HorizontalAlignment','center');
      | 
      | 
      | port_label('input',1,'Q1');
      | port_label('input',2,'Q2');
      | port_label('output',1,'Qe');
  Terminator : Terminator
  To File : ToFile  Filename=output.mat
  To Workspace1 : ToWorkspace  VariableName=yout  SampleTime=-1
  WWTP : Subsystem  mask(WWTP){REmin=[0.85 0.8 0.75], Cemax=[5 .2 .5], n_comp=CD2_get_substances_count}
      mask prompts: REmin "Removal Efficiency REmin [-]"; Cemax "Maximum effluent concnetration Cemax [g/m³]"; n_comp "Number of Components ()"
      mask help:
      | Simple WWTP model. Inflow given is treated according to userdefined maximum concnetration limits and treatment efficiencies.
      |
      | Function used:
      | CD1_sfun_WWTP.m
      mask init:
      | % reading the toplevel systems' name 
      | % --> Plant file name;
      | tls=bdroot(gcb); 
      | % Obtaining the fixed sampling time
      | t_samp_char=get_param(tls, 'FixedStep');
      | % Convertion to numeric value
      | tstep = str2num(t_samp_char); 
      | 
      | RE=REmin;
      | for i=1:n_comp
      | 	if REmin(i) < 0 
      | 		RE(i)=0;
      | 		fprintf('WARNING, Block WWTP:  Removal efficientc of component %u has set to 0, User input REmin <0 \n',i);
      | 	elseif REmin(i) > 1
      | 		RE(i)=1;
      | 		fprintf('WARNING, Block WWTP:  Removal efficientc of component %u has set to 1, User input REmin >1 \n',i);
      | 	else
      | 		RE(i)=REmin(i);
      | 	end
      | end
      | fprintf('\n');
      mask Display:
      | plot(0,0,100,100);
      | plot( [20,50,50,20,20],[30,30,55,55,30], [60,80,70,60],[60,60,20,60], [50, 65],[40,40] );
      | 
      | 
      | text(50,80,'WWTP','HorizontalAlignment','center');
      | text(50,20,'--','HorizontalAlignment','center');
      | 
      | 
      | port_label('input',1,'Qi');
      | port_label('output',1,'Qw');
  x,V1 : Selector  InputPortWidth=3*14  IndexOptions=Index vector (dialog)  Indices=(1:14)  OutputSizes=1
  wires:
  Retention Sewer/1(Qro) -> Retention Sewer/1(Qri)
  Retention Catchment CSS/1(Qro) -> Retention Catchment CSS/1(Qri)
  Retention Catchment SSS/1(Qr) -> Retention Catchment SSS/1(Qri)

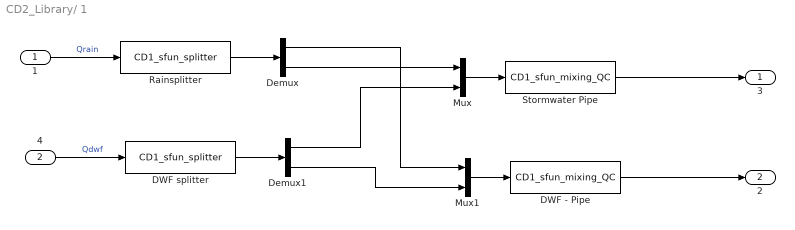
== system CD2_Library/ 1 ==
  " 1" : Inport
  " 4" : Inport  Port=2
  DWF - Pipe : S-Function  FunctionName=CD1_sfun_mixing_QC  Parameters=n_comp,tstep  SFunctionDeploymentMode=off  EnableBusSupport=off
  DWF splitter : S-Function  FunctionName=CD1_sfun_splitter  Parameters=n_comp,values_dwf,mode_dwf,tstep  SFunctionDeploymentMode=off  EnableBusSupport=off
  Demux : Demux  Outputs=2
  Demux1 : Demux  Outputs=2
  Mux : Mux  Inputs=2
  Mux1 : Mux  Inputs=2
  Rainsplitter : S-Function  FunctionName=CD1_sfun_splitter  Parameters=n_comp,values_rain,mode_rain,tstep  SFunctionDeploymentMode=off  EnableBusSupport=off
  Stormwater Pipe : S-Function  FunctionName=CD1_sfun_mixing_QC  Parameters=n_comp,tstep  SFunctionDeploymentMode=off  EnableBusSupport=off
  " 3" : Outport
  " 2" : Outport  Port=2
  wires:
  " 1"/1 -> Rainsplitter/1  "Qrain"
  Rainsplitter/1 -> Demux/1
  " 4"/1 -> DWF splitter/1  "Qdwf"
  DWF splitter/1 -> Demux1/1
  Mux/1 -> Stormwater Pipe/1
  Demux/2 -> Mux/1
  Demux1/1 -> Mux/2
  Mux1/1 -> DWF - Pipe/1
  Demux/1 -> Mux1/1
  Demux1/2 -> Mux1/2
  DWF - Pipe/1 -> " 2"/1
  Stormwater Pipe/1 -> " 3"/1

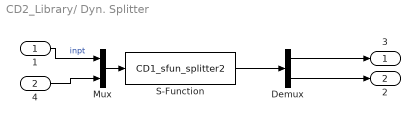
== system CD2_Library/ Dyn. Splitter ==
  " 1" : Inport
  " 4" : Inport  Port=2
  Demux : Demux  Outputs=2
  Mux : Mux  Inputs=[CD2_get_substance_count(subs_vect),n_comp+1]
  S-Function : S-Function  FunctionName=CD1_sfun_splitter2  Parameters=n_comp,mode,tstep  SFunctionDeploymentMode=off  EnableBusSupport=off
  " 3" : Outport
  " 2" : Outport  Port=2
  wires:
  Demux/2 -> " 2"/1
  Demux/1 -> " 3"/1
  S-Function/1 -> Demux/1
  Mux/1 -> S-Function/1
  " 1"/1 -> Mux/1  "inpt"
  " 4"/1 -> Mux/2

== system CD2_Library/ Hydropower 01 ==
  qa [m³/s] ... additional flow : Inport
  q0 [m³/s] ... baseflow : Inport  Port=2
  Mux : Mux  Inputs=2
  S-Function2 : S-Function  FunctionName=CD1_sfun_hydropower  Parameters=n_comp,C_Stream,tstep  SFunctionDeploymentMode=off  EnableBusSupport=off
  Runoff vector Q,C : Outport
  wires:
  Mux/1 -> S-Function2/1
  S-Function2/1 -> Runoff vector Q,C/1
  q0 [m³/s] ... baseflow/1 -> Mux/2
  qa [m³/s] ... additional flow/1 -> Mux/1

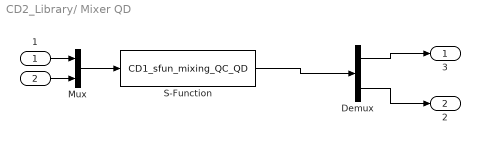
== system CD2_Library/ Mixer QD ==
  " 1" : Inport
  " " : Inport  Port=2
  Demux : Demux  Outputs=[ (n_comp+1) (n_comp+1)]
  Mux : Mux  Inputs=2
  S-Function : S-Function  FunctionName=CD1_sfun_mixing_QC_QD  Parameters=n_comp,tstep,Cmcl  SFunctionDeploymentMode=off  EnableBusSupport=off
  " 3" : Outport
  " 2" : Outport  Port=2
  wires:
  " "/1 -> Mux/2
  " 1"/1 -> Mux/1
  Mux/1 -> S-Function/1
  Demux/1 -> " 3"/1
  Demux/2 -> " 2"/1
  S-Function/1 -> Demux/1

== system CD2_Library/ASM WWTP ==
  " 1" : Inport
  Demux : Demux  Outputs=[n_comp+1,11]
  S-Function : S-Function  FunctionName=CD2_sfun_rumba_wwtp  Parameters=frac,n_comp,wwtpfile,dtwwtp,tstep  SFunctionDeploymentMode=off  EnableBusSupport=off
  " 3" : Outport
  " 2" : Outport  Port=2
  wires:
  Demux/1 -> " 3"/1
  Demux/2 -> " 2"/1
  S-Function/1 -> Demux/1
  " 1"/1 -> S-Function/1

== system CD2_Library/CD Parameters ==

== system CD2_Library/CD02-User Manual ==

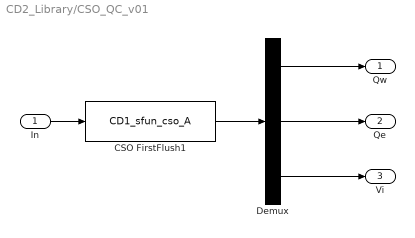
== system CD2_Library/CSO_QC_v01 ==
  In : Inport
  CSO FirstFlush1 : S-Function  FunctionName=CD1_sfun_cso_A  Parameters=Vmax,Qemax,n_comp,tstep  SFunctionDeploymentMode=off  EnableBusSupport=off
  Demux : Demux  Outputs=[ (n_comp+1) (n_comp+1) (n_comp+1)]
  Qw : Outport
  Qe : Outport  Port=2
  Vi : Outport  Port=3
  wires:
  In/1 -> CSO FirstFlush1/1
  CSO FirstFlush1/1 -> Demux/1
  Demux/1 -> Qw/1
  Demux/2 -> Qe/1
  Demux/3 -> Vi/1

== system CD2_Library/CSO_QC_v02 ==
  In : Inport
  CSO FirstFlush1 : S-Function  FunctionName=CD1_sfun_cso_B  Parameters=Vmax,Qemax,n_comp,n_sed,tstep  SFunctionDeploymentMode=off  EnableBusSupport=off
  Demux : Demux  Outputs=[ (n_comp+1) (n_comp+1) (n_comp+1)]
  Qw : Outport
  Qe : Outport  Port=2
  Vi : Outport  Port=3
  wires:
  In/1 -> CSO FirstFlush1/1
  CSO FirstFlush1/1 -> Demux/1
  Demux/1 -> Qw/1
  Demux/2 -> Qe/1
  Demux/3 -> Vi/1

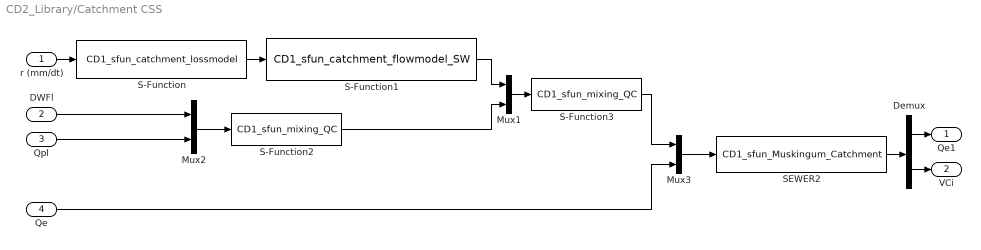
== system CD2_Library/Catchment CSS ==
  r (mm/dt) : Inport
  DWFl : Inport  Port=2
  Qpl : Inport  Port=3
  Qe : Inport  Port=4
  Demux : Demux  Outputs=[n_comp+1,N*(n_comp+1)]
  Mux1 : Mux  Inputs=[n_comp+1,n_comp+1]
  Mux2 : Mux  Inputs=[n_comp+1,n_comp+1]
  Mux3 : Mux  Inputs=[n_comp+1,n_comp+1]
  S-Function : S-Function  FunctionName=CD1_sfun_catchment_lossmodel  Parameters=initloss,permloss,rfcoeff  SFunctionDeploymentMode=off  EnableBusSupport=off
  S-Function1 : S-Function  FunctionName=CD1_sfun_catchment_flowmodel_SW  Parameters=area,n_comp,Rain_C,tstep  SFunctionDeploymentMode=off  EnableBusSupport=off
  S-Function2 : S-Function  FunctionName=CD1_sfun_mixing_QC  Parameters=n_comp,tstep  SFunctionDeploymentMode=off  EnableBusSupport=off
  S-Function3 : S-Function  FunctionName=CD1_sfun_mixing_QC  Parameters=n_comp,tstep  SFunctionDeploymentMode=off  EnableBusSupport=off
  SEWER2 : S-Function  FunctionName=CD1_sfun_Muskingum_Catchment  Parameters=tstep, CX, CY, n_comp,N  SFunctionDeploymentMode=off  EnableBusSupport=off
  Qe1 : Outport
  VCi : Outport  Port=2
  wires:
  S-Function1/1 -> Mux1/1
  Mux2/1 -> S-Function2/1
  r (mm/dt)/1 -> S-Function/1
  S-Function/1 -> S-Function1/1
  Qpl/1 -> Mux2/2
  DWFl/1 -> Mux2/1
  S-Function2/1 -> Mux1/2
  Mux1/1 -> S-Function3/1
  S-Function3/1 -> Mux3/1
  Qe/1 -> Mux3/2
  Mux3/1 -> SEWER2/1
  SEWER2/1 -> Demux/1
  Demux/1 -> Qe1/1
  Demux/2 -> VCi/1

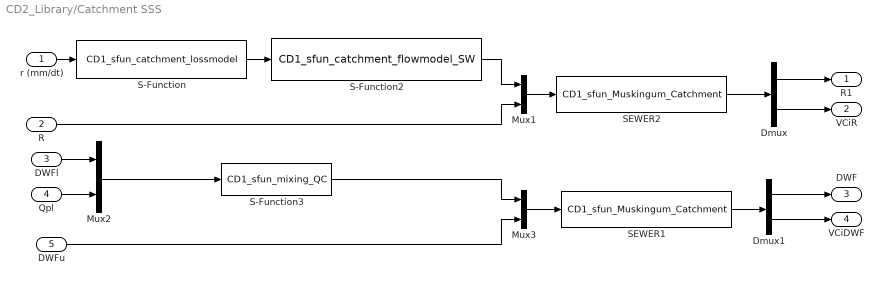
== system CD2_Library/Catchment SSS ==
  r (mm/dt) : Inport
  R : Inport  Port=2
  DWFl : Inport  Port=3
  Qpl : Inport  Port=4
  DWFu : Inport  Port=5
  Dmux : Demux  Outputs=[n_comp+1,N*(n_comp+1)]
  Dmux1 : Demux  Outputs=[n_comp+1,N*(n_comp+1)]
  Mux1 : Mux  Inputs=[n_comp+1,n_comp+1]
  Mux2 : Mux  Inputs=[n_comp+1,n_comp+1]
  Mux3 : Mux  Inputs=[n_comp+1,n_comp+1]
  S-Function : S-Function  FunctionName=CD1_sfun_catchment_lossmodel  Parameters=initloss,permloss,rfcoeff  SFunctionDeploymentMode=off  EnableBusSupport=off
  S-Function2 : S-Function  FunctionName=CD1_sfun_catchment_flowmodel_SW  Parameters=area,n_comp,Rain_C,tstep  SFunctionDeploymentMode=off  EnableBusSupport=off
  S-Function3 : S-Function  FunctionName=CD1_sfun_mixing_QC  Parameters=n_comp,tstep  SFunctionDeploymentMode=off  EnableBusSupport=off
  SEWER1 : S-Function  FunctionName=CD1_sfun_Muskingum_Catchment  Parameters=tstep, CX, CY, n_comp,N  SFunctionDeploymentMode=off  EnableBusSupport=off
  SEWER2 : S-Function  FunctionName=CD1_sfun_Muskingum_Catchment  Parameters=tstep, CX, CY, n_comp,N  SFunctionDeploymentMode=off  EnableBusSupport=off
  R1 : Outport
  VCiR : Outport  Port=2
  "DWF " : Outport  Port=3
  VCiDWF : Outport  Port=4
  wires:
  S-Function/1 -> S-Function2/1
  r (mm/dt)/1 -> S-Function/1
  DWFl/1 -> Mux2/1
  R/1 -> Mux1/2
  S-Function2/1 -> Mux1/1
  Mux1/1 -> SEWER2/1
  Mux3/1 -> SEWER1/1
  SEWER2/1 -> Dmux/1
  Dmux/1 -> R1/1
  SEWER1/1 -> Dmux1/1
  Dmux1/1 -> "DWF "/1
  Dmux/2 -> VCiR/1
  Dmux1/2 -> VCiDWF/1
  Qpl/1 -> Mux2/2
  Mux2/1 -> S-Function3/1
  S-Function3/1 -> Mux3/1
  DWFu/1 -> Mux3/2

== system CD2_Library/Flowread ==
  flowread : S-Function  FunctionName=CD1_sfun_flowread  Parameters=dtype,crep,table,tstep  SFunctionDeploymentMode=off  EnableBusSupport=off
  out_1 : Outport
  wires:
  flowread/1 -> out_1/1

== system CD2_Library/LOGO ==

== system CD2_Library/LOGO1 ==
